simulink model "MCU_Stateflow_Analog"  (R2022b)
settings: Solver=FixedStepDiscrete  StartTime=0.0  StopTime=inf  FixedStep=0.002  RelTol=1e-3
undefined symbols (not defined in the file): ANALOG, cAgeingMode, cCurrentLoopMode, cNoneMode, cParaRecogMode, cSingleBoardMode, cSpeedLoopMode, cTorqueLoopMode, cVvvfOpenMode, FAULT, POWER_ON, STANDBY, TESTBED, VEHICLE, WORKING
libraries: simulink x9, SignalEditorBlockLib x1
(part 1 of 4)
Description:
  | 1、增加Analog模式
  | 2、增加转速选择
settings Model: DataDictionary=MCU_Stateflow_Datadictionary_objects.sldd  Creator=ZYH  LastModifiedBy=ZYH
settings OptimizationCC: DefaultParameterBehavior=Inlined  EnhancedBackFolding=on  PassReuseOutputArgsAs=Individual arguments  ZeroExternalMemoryAtStartup=off  ZeroInternalMemoryAtStartup=off  OptimizeBlockOrder=speed  DifferentSizesBufferReuse=on  OptimizationCustomize=off  EfficientTunableParamExpr=on
settings DebuggingCC: ParameterTunabilityLossMsg=error
settings ModelReferenceCC: ModelReferenceNumInstancesAllowed=Single
settings SFSimCC: MATLABDynamicMemAlloc=off
settings RTWCC: Description=Embedded Coder  SystemTargetFile=ert.tlc  GenCodeOnly=on  TemplateMakefile=ert_default_tmf
settings CodeAppCC: IgnoreCustomStorageClasses=off  OperatorAnnotations=on  SimulinkDataObjDesc=on  SFDataObjDesc=on  CustomSymbolStrGlobalVar=$N$M  CustomSymbolStrType=$N$M_T  CustomSymbolStrFcn=$N$M$F
settings ERTTargetCC: TargetLangStandard=C99 (ISO)  GenerateSampleERTMain=on  InlinedParameterPlacement=NonHierarchical  MultiInstanceErrorCode=None  RootIOFormat=Structure reference  ERTCustomFileTemplate=example_file_process.tlc

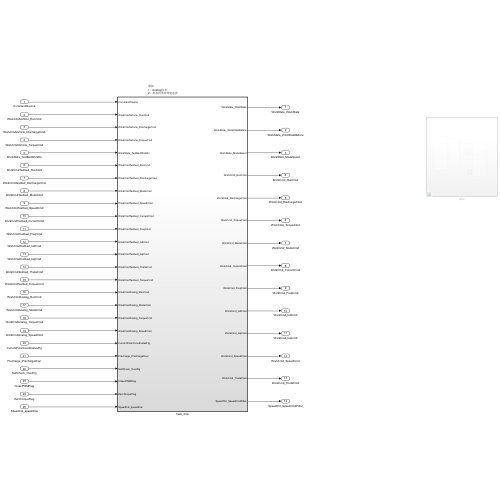
[thumbnail: Simulink's stored preview of the top-level diagram]
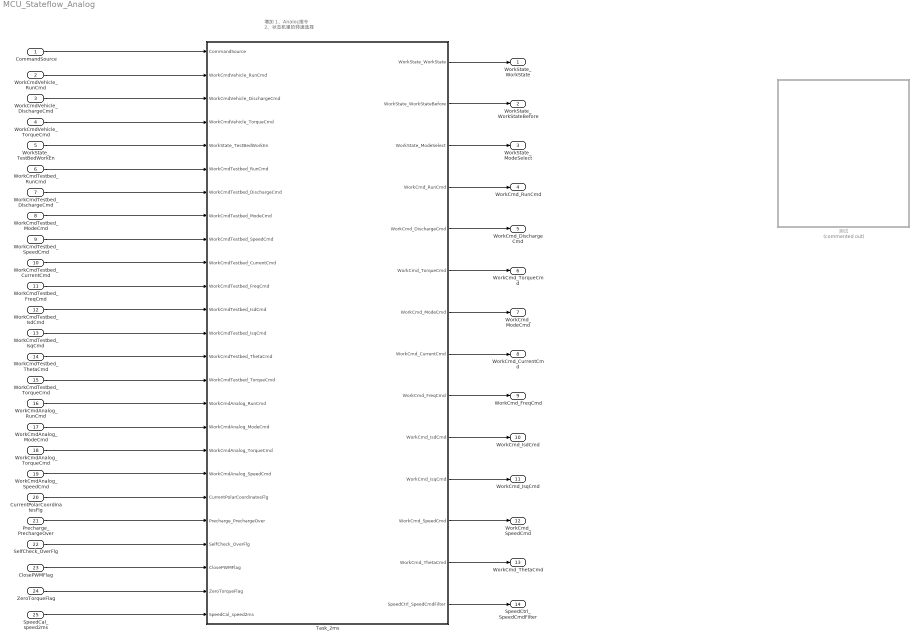
== system MCU_Stateflow_Analog ==
  note: 增加
      | 1、Analog指令
      | 2、状态机里的转速选择
  CommandSource : Inport
  WorkCmdVehicle_RunCmd : Inport  Port=2
  WorkCmdVehicle_DischargeCmd : Inport  Port=3
  WorkCmdVehicle_TorqueCmd : Inport  Port=4
  WorkState_TestBedWorkEn : Inport  Port=5
  WorkCmdTestbed_RunCmd : Inport  Port=6
  WorkCmdTestbed_DischargeCmd : Inport  Port=7
  WorkCmdTestbed_ModeCmd : Inport  Port=8
  WorkCmdTestbed_SpeedCmd : Inport  Port=9
  WorkCmdTestbed_CurrentCmd : Inport  Port=10
  WorkCmdTestbed_FreqCmd : Inport  Port=11
  WorkCmdTestbed_IsdCmd : Inport  Port=12
  WorkCmdTestbed_IsqCmd : Inport  Port=13
  WorkCmdTestbed_ThetaCmd : Inport  Port=14
  WorkCmdTestbed_TorqueCmd : Inport  Port=15
  WorkCmdAnalog_RunCmd : Inport  Port=16
  WorkCmdAnalog_ModeCmd : Inport  Port=17
  WorkCmdAnalog_TorqueCmd : Inport  Port=18
  WorkCmdAnalog_SpeedCmd : Inport  Port=19
  CurrentPolarCoordinatesFlg : Inport  Port=20
  Precharge_PrechargeOver : Inport  Port=21
  SelfCheck_OverFlg : Inport  Port=22
  ClosePWMFlag : Inport  Port=23
  ZeroTorqueFlag : Inport  Port=24
  SpeedCal_speed2ms : Inport  Port=25
  Task_2ms : Subsystem  TreatAsAtomicUnit=on
      settings: RTWSystemCode=Inline
  测试 : Subsystem  Commented=on
  WorkState_WorkState : Outport
  WorkState_WorkStateBefore : Outport  Port=2
  WorkState_ModeSelect : Outport  Port=3
  WorkCmd_RunCmd : Outport  Port=4
  WorkCmd_DischargeCmd : Outport  Port=5
  WorkCmd_TorqueCmd : Outport  Port=6
  WorkCmd_ModeCmd : Outport  Port=7
  WorkCmd_CurrentCmd : Outport  Port=8
  WorkCmd_FreqCmd : Outport  Port=9
  WorkCmd_IsdCmd : Outport  Port=10
  WorkCmd_IsqCmd : Outport  Port=11
  WorkCmd_SpeedCmd : Outport  Port=12
  WorkCmd_ThetaCmd : Outport  Port=13
  SpeedCtrl_SpeedCmdFilter : Outport  Port=14
  wires:
  CommandSource/1 -> Task_2ms/1(CommandSource)
  WorkCmdVehicle_RunCmd/1 -> Task_2ms/2(WorkCmdVehicle_RunCmd)
  WorkCmdVehicle_DischargeCmd/1 -> Task_2ms/3(WorkCmdVehicle_DischargeCmd)
  WorkState_TestBedWorkEn/1 -> Task_2ms/5(WorkState_TestBedWorkEn)
  WorkCmdTestbed_RunCmd/1 -> Task_2ms/6(WorkCmdTestbed_RunCmd)
  WorkCmdTestbed_DischargeCmd/1 -> Task_2ms/7(WorkCmdTestbed_DischargeCmd)
  WorkCmdTestbed_ModeCmd/1 -> Task_2ms/8(WorkCmdTestbed_ModeCmd)
  WorkCmdTestbed_SpeedCmd/1 -> Task_2ms/9(WorkCmdTestbed_SpeedCmd)
  WorkCmdTestbed_CurrentCmd/1 -> Task_2ms/10(WorkCmdTestbed_CurrentCmd)
  WorkCmdTestbed_FreqCmd/1 -> Task_2ms/11(WorkCmdTestbed_FreqCmd)
  WorkCmdTestbed_IsdCmd/1 -> Task_2ms/12(WorkCmdTestbed_IsdCmd)
  WorkCmdTestbed_IsqCmd/1 -> Task_2ms/13(WorkCmdTestbed_IsqCmd)
  WorkCmdTestbed_ThetaCmd/1 -> Task_2ms/14(WorkCmdTestbed_ThetaCmd)
  WorkCmdVehicle_TorqueCmd/1 -> Task_2ms/4(WorkCmdVehicle_TorqueCmd)
  WorkCmdTestbed_TorqueCmd/1 -> Task_2ms/15(WorkCmdTestbed_TorqueCmd)
  CurrentPolarCoordinatesFlg/1 -> Task_2ms/20(CurrentPolarCoordinatesFlg)
  Precharge_PrechargeOver/1 -> Task_2ms/21(Precharge_PrechargeOver)
  ClosePWMFlag/1 -> Task_2ms/23(ClosePWMFlag)
  ZeroTorqueFlag/1 -> Task_2ms/24(ZeroTorqueFlag)
  Task_2ms/1(WorkState_WorkState) -> WorkState_WorkState/1
  Task_2ms/2(WorkState_WorkStateBefore) -> WorkState_WorkStateBefore/1
  Task_2ms/3(WorkState_ModeSelect) -> WorkState_ModeSelect/1
  Task_2ms/4(WorkCmd_RunCmd) -> WorkCmd_RunCmd/1
  Task_2ms/5(WorkCmd_DischargeCmd) -> WorkCmd_DischargeCmd/1
  Task_2ms/6(WorkCmd_TorqueCmd) -> WorkCmd_TorqueCmd/1
  Task_2ms/7(WorkCmd_ModeCmd) -> WorkCmd_ModeCmd/1
  Task_2ms/8(WorkCmd_CurrentCmd) -> WorkCmd_CurrentCmd/1
  Task_2ms/9(WorkCmd_FreqCmd) -> WorkCmd_FreqCmd/1
  Task_2ms/10(WorkCmd_IsdCmd) -> WorkCmd_IsdCmd/1
  Task_2ms/11(WorkCmd_IsqCmd) -> WorkCmd_IsqCmd/1
  Task_2ms/12(WorkCmd_SpeedCmd) -> WorkCmd_SpeedCmd/1
  Task_2ms/13(WorkCmd_ThetaCmd) -> WorkCmd_ThetaCmd/1
  SelfCheck_OverFlg/1 -> Task_2ms/22(SelfCheck_OverFlg)
  WorkCmdAnalog_RunCmd/1 -> Task_2ms/16(WorkCmdAnalog_RunCmd)
  WorkCmdAnalog_ModeCmd/1 -> Task_2ms/17(WorkCmdAnalog_ModeCmd)
  WorkCmdAnalog_TorqueCmd/1 -> Task_2ms/18(WorkCmdAnalog_TorqueCmd)
  WorkCmdAnalog_SpeedCmd/1 -> Task_2ms/19(WorkCmdAnalog_SpeedCmd)
  SpeedCal_speed2ms/1 -> Task_2ms/25(SpeedCal_speed2ms)
  Task_2ms/14(SpeedCtrl_SpeedCmdFilter) -> SpeedCtrl_SpeedCmdFilter/1

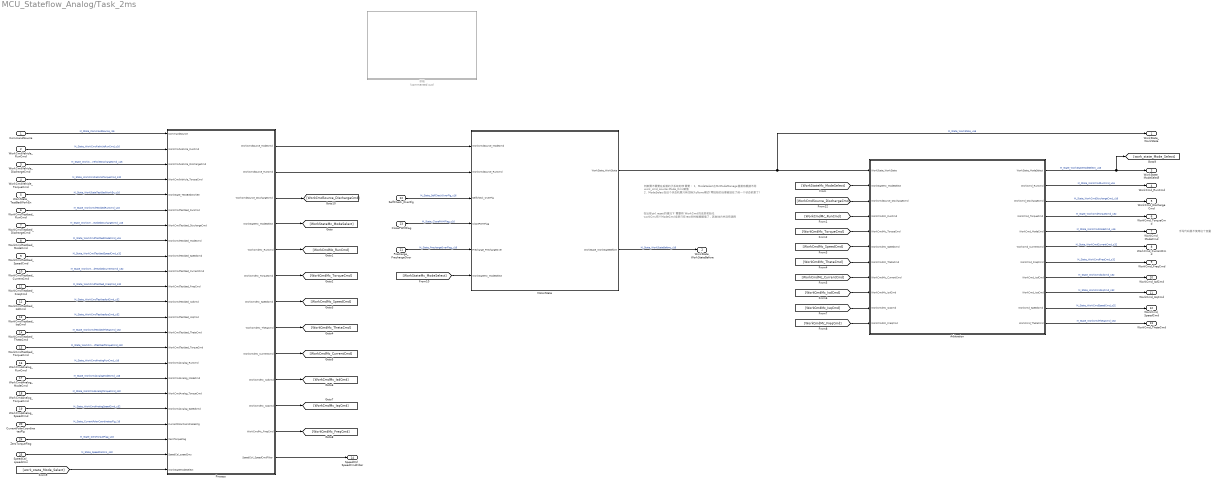
== system MCU_Stateflow_Analog/Task_2ms ==
  note: 手写代码里不使用这个变量
  note: 在出现ctrl_reset的情况下
      | 需要将 WorkCmd 的成员初始化
      | workCmd有个ModeCmd成员只在rest的时候被赋值了，其他地方并没有调用
  note: 判断需不需要在后面的子系统处理
      |
      | 需要：
      | 1、ModeSelect在McModeManage里面有根据不同 work_cmd_source.Mode_Cmd赋值
      | 2、ModeSelect在这个状态机里只有切换为cNone模式(零扭矩的处理被放在了前一个状态机里了)
  CommandSource : Inport
  WorkCmdVehicle_RunCmd : Inport  Port=2
  WorkCmdVehicle_DischargeCmd : Inport  Port=3
  WorkCmdVehicle_TorqueCmd : Inport  Port=4
  WorkState_TestBedWorkEn : Inport  Port=5
  WorkCmdTestbed_RunCmd : Inport  Port=6
  WorkCmdTestbed_DischargeCmd : Inport  Port=7
  WorkCmdTestbed_ModeCmd : Inport  Port=8
  WorkCmdTestbed_SpeedCmd : Inport  Port=9
  WorkCmdTestbed_CurrentCmd : Inport  Port=10
  WorkCmdTestbed_FreqCmd : Inport  Port=11
  WorkCmdTestbed_IsdCmd : Inport  Port=12
  WorkCmdTestbed_IsqCmd : Inport  Port=13
  WorkCmdTestbed_ThetaCmd : Inport  Port=14
  WorkCmdTestbed_TorqueCmd : Inport  Port=15
  WorkCmdAnalog_RunCmd : Inport  Port=16
  WorkCmdAnalog_ModeCmd : Inport  Port=17
  WorkCmdAnalog_TorqueCmd : Inport  Port=18
  WorkCmdAnalog_SpeedCmd : Inport  Port=19
  CurrentPolarCoordinatesFlg : Inport  Port=20
  Precharge_PrechargeOver : Inport  Port=21
  SelfCheck_OverFlg : Inport  Port=22
  ClosePWMFlag : Inport  Port=23
  ZeroTorqueFlag : Inport  Port=24
  SpeedCal_speed2ms : Inport  Port=25
  Arbitration : Subsystem  TreatAsAtomicUnit=on
  MotorState : Stateflow chart  TreatAsAtomicUnit=on
      settings: RTWSystemCode=Reusable function  PortSchema="{\"entries\":[{\"content\":{\"sides\":[{\"content\":{\"connectorIds\":[\"In4\",\"In3\",\"In1\",\"In2\",\"In5\",\"In6\"]},\"type\":\"ConnectorPlacement.EquallySpacedRectSide\",\"uuid\":\"e0adab7d-9c82-44fd-b38c-331bb9d71454\"},{\"content\":{\"connectorIds\":[\"Out1\",\"Out2\"],\"side\":\"RIGHT\"},\"type\":\"ConnectorPlacement.EquallySpacedRectSide\",\"uuid\":\"98ad1acc-debf-46f0-91aa-4bd2062f60b6\"},{\"content\":{\"connectorIds\":[],\"side\":\"TOP\"},\"type\":\"ConnectorPlacement.EquallySpacedRectSide\",\"uuid\":\"a7c2d312-245c-4ce1-bea5-1bac95c515f1\"},{\"content\":{\"connectorIds\":[],\"side\":\"BOTTOM\"},\"type\":\"ConnectorPlacement.EquallySpacedRectSide\",\"uuid\":\"175f3b6b-1019-4e6e-83d9-bf4c82f74bc8\"}]},\"type\":\"ConnectorPlacement.EquallySpacedConnector\",\"uuid\":\"df312d8c-c57e-4b1a-958b-330641c1b4d1\"}],\"packageUris\":[\"http://schema.mathworks.com/mf0/Connector/R2020b\"],\"version\":\"1.0\"}"
  Process : Subsystem  TreatAsAtomicUnit=on
  草稿 : Subsystem  Commented=on
  WorkState_WorkState : Outport
  WorkState_WorkStateBefore : Outport  Port=2
  WorkState_ModeSelect : Outport  Port=3
  WorkCmd_RunCmd : Outport  Port=4
  WorkCmd_DischargeCmd : Outport  Port=5
  WorkCmd_TorqueCmd : Outport  Port=6
  WorkCmd_ModeCmd : Outport  Port=7
  WorkCmd_CurrentCmd : Outport  Port=8
  WorkCmd_FreqCmd : Outport  Port=9
  WorkCmd_IsdCmd : Outport  Port=10
  WorkCmd_IsqCmd : Outport  Port=11
  WorkCmd_SpeedCmd : Outport  Port=12
  WorkCmd_ThetaCmd : Outport  Port=13
  SpeedCtrl_SpeedCmdFilter : Outport  Port=14
  wires:
  MotorState/1(WorkState_WorkState) -> WorkState_WorkState/1, Arbitration/1(WorkState_WorkState)  "M_State_WorkState_u16"
  [WorkStateMc_ModeSelect] -> Arbitration/2(WorkStateMc_ModeSelect)
  [WorkCmdMc_RunCmd] -> Arbitration/4(WorkCmdMc_RunCmd)
  [WorkCmdMc_TorqueCmd] -> Arbitration/5(WorkCmdMc_TorqueCmd)
  [WorkCmdMc_SpeedCmd] -> Arbitration/6(WorkCmdMc_SpeedCmd)
  [WorkCmdMc_ThetaCmd] -> Arbitration/7(WorkCmdMc_ThetaCmd)
  [WorkCmdMc_CurrentCmd] -> Arbitration/8(WorkCmdMc_CurrentCmd)
  [WorkCmdMc_IsdCmd] -> Arbitration/9(WorkCmdMc_IsdCmd)
  [WorkCmdMc_IsqCmd] -> Arbitration/10(WorkCmdMc_IsqCmd)
  [WorkCmdMc_FreqCmd] -> Arbitration/11(WorkCmdMc_FreqCmd)
  Precharge_PrechargeOver/1 -> MotorState/5(Precharge_PrechargeOver)  "M_State_PrechargeOverFlag_u16"
  MotorState/2(WorkState_WorkStateBefore) -> WorkState_WorkStateBefore/1  "M_State_WorkStateBefore_u16"
  Process/8(WorkCmdMc_ThetaCmd) -> [WorkCmdMc_ThetaCmd]
  Process/9(WorkCmdMc_CurrentCmd) -> [WorkCmdMc_CurrentCmd]
  Process/7(WorkCmdMc_SpeedCmd) -> [WorkCmdMc_SpeedCmd]
  Process/12(WorkCmdMc_FreqCmd) -> [WorkCmdMc_FreqCmd]
  Process/5(WorkCmdMc_RunCmd) -> [WorkCmdMc_RunCmd]
  Process/10(WorkCmdMc_IsdCmd) -> [WorkCmdMc_IsdCmd]
  Process/11(WorkCmdMc_IsqCmd) -> [WorkCmdMc_IsqCmd]
  Process/6(WorkCmdMc_TorqueCmd) -> [WorkCmdMc_TorqueCmd]
  Process/4(WorkStateMc_ModeSelect) -> [WorkStateMc_ModeSelect]
  CommandSource/1 -> Process/1(CommandSource)  "M_State_CommandSource_i16"
  WorkCmdVehicle_RunCmd/1 -> Process/2(WorkCmdVehicle_RunCmd)  "M_State_WorkCmdVehicleRunCmd_u16"
  WorkCmdVehicle_DischargeCmd/1 -> Process/3(WorkCmdVehicle_DischargeCmd)  "M_State_WorkCmdVehicleDischargeCmd_u16"
  WorkState_TestBedWorkEn/1 -> Process/5(WorkState_TestBedWorkEn)  "M_State_WorkStateTestBedWorkEn_u16"
  WorkCmdTestbed_RunCmd/1 -> Process/6(WorkCmdTestbed_RunCmd)  "M_State_WorkCmdTestbedRunCmd_u16"
  WorkCmdTestbed_DischargeCmd/1 -> Process/7(WorkCmdTestbed_DischargeCmd)  "M_State_WorkCmdTestbedDischargeCmd_u16"
  WorkCmdTestbed_ModeCmd/1 -> Process/8(WorkCmdTestbed_ModeCmd)  "M_State_WorkCmdTestbedModeCmd_u16"
  WorkCmdTestbed_SpeedCmd/1 -> Process/9(WorkCmdTestbed_SpeedCmd)  "M_State_WorkCmdTestbedSpeedCmd_s32"
  WorkCmdTestbed_CurrentCmd/1 -> Process/10(WorkCmdTestbed_CurrentCmd)  "M_State_WorkCmdTestbedCurrentCmd_s32"
  WorkCmdTestbed_FreqCmd/1 -> Process/11(WorkCmdTestbed_FreqCmd)  "M_State_WorkCmdTestbed_FreqCmd_s32"
  WorkCmdTestbed_IsdCmd/1 -> Process/12(WorkCmdTestbed_IsdCmd)  "M_State_WorkCmdTestbedIsdCmd_s32"
  WorkCmdTestbed_IsqCmd/1 -> Process/13(WorkCmdTestbed_IsqCmd)  "M_State_WorkCmdTestbedIsqCmd_s32"
  WorkCmdTestbed_ThetaCmd/1 -> Process/14(WorkCmdTestbed_ThetaCmd)  "M_State_WorkCmdTestbedThetaCmd_s32"
  WorkCmdVehicle_TorqueCmd/1 -> Process/4(WorkCmdVehicle_TorqueCmd)  "M_State_WorkCmdVehicleTorqueCmd_s32"
  WorkCmdTestbed_TorqueCmd/1 -> Process/15(WorkCmdTestbed_TorqueCmd)  "M_State_WorkCmdTestbedTorqueCmd_s32"
  CurrentPolarCoordinatesFlg/1 -> Process/20(CurrentPolarCoordinatesFlg)  "M_State_CurrentPolarCoordinatesFlg_i16"
  ZeroTorqueFlag/1 -> Process/21(ZeroTorqueFlag)  "M_State_ZeroTorqueFlag_u16"
  Process/1(WorkCmdSource_ModeCmd) -> MotorState/4(WorkCmdSource_ModeCmd)
  Process/2(WorkCmdSource_RunCmd) -> MotorState/3(WorkCmdSource_RunCmd)
  Arbitration/1(WorkState_ModeSelect) -> WorkState_ModeSelect/1, [work_state_Mode_Select]  "M_State_WorkStateModeSelect_u16"
  Arbitration/2(WorkCmd_RunCmd) -> WorkCmd_RunCmd/1  "M_State_WorkCmdRunCmd_u16"
  Arbitration/3(WorkCmd_DischargeCmd) -> WorkCmd_DischargeCmd/1  "M_State_WorkCmdDischargeCmd_u16"
  Arbitration/4(WorkCmd_TorqueCmd) -> WorkCmd_TorqueCmd/1  "M_State_WorkCmdTorqueCmd_s32"
  Arbitration/5(WorkCmd_ModeCmd) -> WorkCmd_ModeCmd/1  "M_State_WorkCmdModeCmd_u16"
  Arbitration/6(WorkCmd_CurrentCmd) -> WorkCmd_CurrentCmd/1  "M_State_WorkCmdCurrentCmd_s32"
  Arbitration/7(WorkCmd_FreqCmd) -> WorkCmd_FreqCmd/1  "M_State_WorkCmdFreqCmd_s32"
  Arbitration/8(WorkCmd_IsdCmd) -> WorkCmd_IsdCmd/1  "M_State_WorkCmdIsdCmd_s32"
  Arbitration/9(WorkCmd_IsqCmd) -> WorkCmd_IsqCmd/1  "M_State_WorkCmdIsqCmd_s32"
  Arbitration/10(WorkCmd_SpeedCmd) -> WorkCmd_SpeedCmd/1  "M_State_WorkCmdSpeedCmd_s32"
  Arbitration/11(WorkCmd_ThetaCmd) -> WorkCmd_ThetaCmd/1  "M_State_WorkCmdThetaCmd_s32"
  SelfCheck_OverFlg/1 -> MotorState/1(SelfCheck_OverFlg)  "M_State_SelfCheckOverFlg_u16"
  ClosePWMFlag/1 -> MotorState/2(ClosePWMFlag)  "M_State_ClosePWMFlag_u16"
  [work_state_Mode_Select] -> Process/23(WorkStateModeSelect)
  [WorkStateMc_ModeSelect] -> MotorState/6(WorkStateMc_ModeSelect)
  WorkCmdAnalog_RunCmd/1 -> Process/16(WorkCmdAnalog_RunCmd)  "M_State_WorkCmdAnalogRunCmd_u16"
  WorkCmdAnalog_ModeCmd/1 -> Process/17(WorkCmdAnalog_ModeCmd)  "M_State_WorkCmdAnalogModeCmd_u16"
  WorkCmdAnalog_TorqueCmd/1 -> Process/18(WorkCmdAnalog_TorqueCmd)  "M_State_WorkCmdAnalogTorqueCmd_s32"
  WorkCmdAnalog_SpeedCmd/1 -> Process/19(WorkCmdAnalog_SpeedCmd)  "M_State_WorkCmdAnalogSpeedCmd_s32"
  SpeedCal_speed2ms/1 -> Process/22(SpeedCal_speed2ms)  "M_State_SpeedCal2ms_s32"
  Process/13(SpeedCtrl_SpeedCmdFilter) -> SpeedCtrl_SpeedCmdFilter/1
  Process/3(WorkCmdSource_DischargeCmd) -> [WorkCmdSource_DischargeCmd]
  [WorkCmdSource_DischargeCmd] -> Arbitration/3(WorkCmdSource_DischargeCmd)

== system MCU_Stateflow_Analog/测试 ==
  Constant : Constant  Commented=on
  Constant1 : Constant  Commented=on  Value=0
  Constant2 : Constant  Commented=on  Value=2
  Constant3 : Constant  Commented=on  Value=200
  Constant4 : Constant  Commented=on
  Constant5 : Constant  Commented=on  Value=0
  Data Type Conversion{,1..5} (6 alike) : DataTypeConversion  Commented=on  SaturateOnIntegerOverflow=off  RndMeth=Floor
  Display : Display  Commented=on
  Display1 : Display  Commented=on
  Signal Editor : SignalEditorBlockLib/Signal Editor  Commented=on  FileName=Inputs.mat  ActiveScenario=Scenario  ActiveSignal=CommandSource  IsBus=off  OutputBusObjectStr=Bus: BusObject  SampleTime=0  Interpolate=off  ZeroCross=off  OutputAfterFinalValue=Setting to zero  Unit=inherit  PreserveSignalName=on
  Task_2ms1 : Subsystem  Commented=on  TreatAsAtomicUnit=on
      settings: RTWSystemCode=Inline
  Task_2ms2 : Subsystem  Commented=on  TreatAsAtomicUnit=on
      settings: RTWSystemCode=Inline
  wires:
  Constant/1 -> Data Type Conversion/1
  Constant3/1 -> Data Type Conversion3/1
  Task_2ms1/1(WorkState_WorkState) -> Display/1
  Data Type Conversion5/1 -> Task_2ms1/24(ZeroTorqueFlag), Task_2ms1/23(ClosePWMFlag)
  Data Type Conversion2/1 -> Task_2ms1/8(WorkCmdTestbed_ModeCmd)
  Data Type Conversion4/1 -> Task_2ms1/22(SelfCheck_OverFlg), Task_2ms1/21(Precharge_PrechargeOver)
  Data Type Conversion3/1 -> Task_2ms1/9(WorkCmdTestbed_SpeedCmd)
  Task_2ms1/12(WorkCmd_SpeedCmd) -> Display1/1
  Constant5/1 -> Data Type Conversion5/1
  Constant4/1 -> Data Type Conversion4/1
  Data Type Conversion1/1 -> Task_2ms1/6(WorkCmdTestbed_RunCmd), Task_2ms1/5(WorkState_TestBedWorkEn)
  Constant1/1 -> Data Type Conversion1/1
  Constant2/1 -> Data Type Conversion2/1
  Data Type Conversion/1 -> Task_2ms1/1(CommandSource)

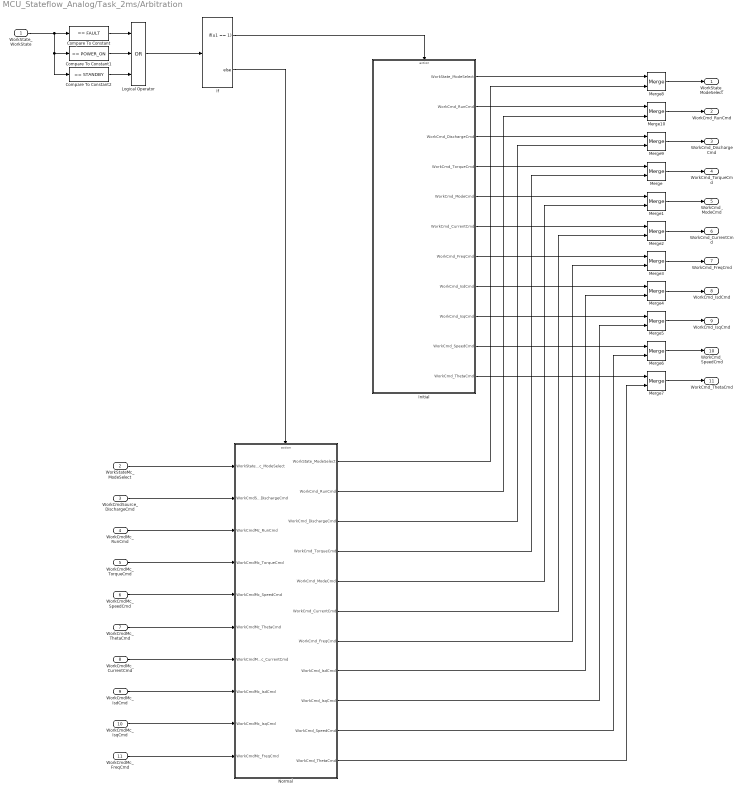
== system MCU_Stateflow_Analog/Task_2ms/Arbitration ==
  WorkState_WorkState : Inport
  WorkStateMc_ModeSelect : Inport  Port=2
  WorkCmdSource_DischargeCmd : Inport  Port=3
  WorkCmdMc_RunCmd : Inport  Port=4
  WorkCmdMc_TorqueCmd : Inport  Port=5
  WorkCmdMc_SpeedCmd : Inport  Port=6
  WorkCmdMc_ThetaCmd : Inport  Port=7
  WorkCmdMc_CurrentCmd : Inport  Port=8
  WorkCmdMc_IsdCmd : Inport  Port=9
  WorkCmdMc_IsqCmd : Inport  Port=10
  WorkCmdMc_FreqCmd : Inport  Port=11
  Compare To Constant : simulink/Logic and Bit Operations/Compare To Constant  relop===  const=FAULT  OutDataTypeStr=boolean
  Compare To Constant1 : simulink/Logic and Bit Operations/Compare To Constant  relop===  const=POWER_ON  OutDataTypeStr=boolean
  Compare To Constant2 : simulink/Logic and Bit Operations/Compare To Constant  relop===  const=STANDBY  OutDataTypeStr=boolean
  If : If  IfExpression=u1 == 1
  Initial : Subsystem  TreatAsAtomicUnit=on
  Logical Operator : Logic  Operator=OR  Inputs=3  AllPortsSameDT=off  OutDataTypeStr=boolean
  Merge{,1..10} (11 alike) : Merge
  Normal : Subsystem  TreatAsAtomicUnit=on
  WorkState_ModeSelect : Outport
  WorkCmd_RunCmd : Outport  Port=2
  WorkCmd_DischargeCmd : Outport  Port=3
  WorkCmd_TorqueCmd : Outport  Port=4
  WorkCmd_ModeCmd : Outport  Port=5
  WorkCmd_CurrentCmd : Outport  Port=6
  WorkCmd_FreqCmd : Outport  Port=7
  WorkCmd_IsdCmd : Outport  Port=8
  WorkCmd_IsqCmd : Outport  Port=9
  WorkCmd_SpeedCmd : Outport  Port=10
  WorkCmd_ThetaCmd : Outport  Port=11
  wires:
  WorkState_WorkState/1 -> Compare To Constant2/1, Compare To Constant1/1, Compare To Constant/1
  Compare To Constant/1 -> Logical Operator/1
  Compare To Constant1/1 -> Logical Operator/2
  Compare To Constant2/1 -> Logical Operator/3
  Logical Operator/1 -> If/1
  If/1 -> Initial/Action
  If/2 -> Normal/Action
  Initial/11(WorkCmd_ThetaCmd) -> Merge7/1
  Initial/10(WorkCmd_SpeedCmd) -> Merge6/1
  Initial/9(WorkCmd_IsqCmd) -> Merge5/1
  Initial/8(WorkCmd_IsdCmd) -> Merge4/1
  Initial/7(WorkCmd_FreqCmd) -> Merge3/1
  Initial/6(WorkCmd_CurrentCmd) -> Merge2/1
  Initial/5(WorkCmd_ModeCmd) -> Merge1/1
  Initial/4(WorkCmd_TorqueCmd) -> Merge/1
  Initial/3(WorkCmd_DischargeCmd) -> Merge9/1
  WorkStateMc_ModeSelect/1 -> Normal/1(WorkStateMc_ModeSelect)
  WorkCmdMc_RunCmd/1 -> Normal/3(WorkCmdMc_RunCmd)
  WorkCmdMc_TorqueCmd/1 -> Normal/4(WorkCmdMc_TorqueCmd)
  WorkCmdMc_SpeedCmd/1 -> Normal/5(WorkCmdMc_SpeedCmd)
  WorkCmdMc_ThetaCmd/1 -> Normal/6(WorkCmdMc_ThetaCmd)
  WorkCmdMc_CurrentCmd/1 -> Normal/7(WorkCmdMc_CurrentCmd)
  WorkCmdMc_IsdCmd/1 -> Normal/8(WorkCmdMc_IsdCmd)
  WorkCmdMc_IsqCmd/1 -> Normal/9(WorkCmdMc_IsqCmd)
  WorkCmdMc_FreqCmd/1 -> Normal/10(WorkCmdMc_FreqCmd)
  Merge/1 -> WorkCmd_TorqueCmd/1
  Merge1/1 -> WorkCmd_ModeCmd/1
  Merge2/1 -> WorkCmd_CurrentCmd/1
  Merge3/1 -> WorkCmd_FreqCmd/1
  Merge4/1 -> WorkCmd_IsdCmd/1
  Merge5/1 -> WorkCmd_IsqCmd/1
  Merge6/1 -> WorkCmd_SpeedCmd/1
  Merge7/1 -> WorkCmd_ThetaCmd/1
  Initial/1(WorkState_ModeSelect) -> Merge8/1
  Merge8/1 -> WorkState_ModeSelect/1
  Initial/2(WorkCmd_RunCmd) -> Merge10/1
  Merge10/1 -> WorkCmd_RunCmd/1
  Merge9/1 -> WorkCmd_DischargeCmd/1
  Normal/1(WorkState_ModeSelect) -> Merge8/2
  Normal/2(WorkCmd_RunCmd) -> Merge10/2
  Normal/3(WorkCmd_DischargeCmd) -> Merge9/2
  Normal/4(WorkCmd_TorqueCmd) -> Merge/2
  Normal/5(WorkCmd_ModeCmd) -> Merge1/2
  Normal/6(WorkCmd_CurrentCmd) -> Merge2/2
  Normal/7(WorkCmd_FreqCmd) -> Merge3/2
  Normal/8(WorkCmd_IsdCmd) -> Merge4/2
  Normal/9(WorkCmd_IsqCmd) -> Merge5/2
  Normal/10(WorkCmd_SpeedCmd) -> Merge6/2
  Normal/11(WorkCmd_ThetaCmd) -> Merge7/2
  WorkCmdSource_DischargeCmd/1 -> Normal/2(WorkCmdSource_DischargeCmd)

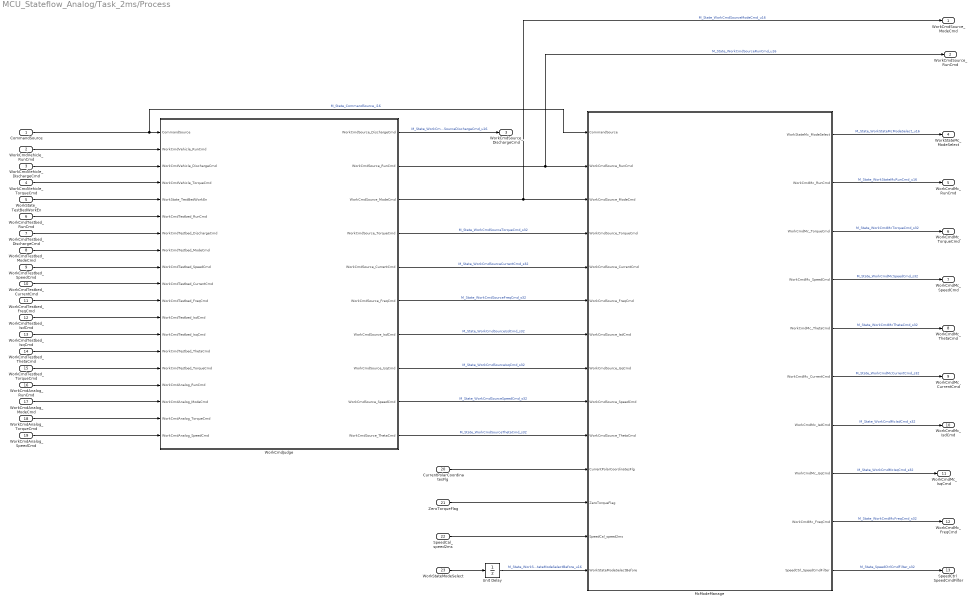
== system MCU_Stateflow_Analog/Task_2ms/Process ==
  CommandSource : Inport
  WorkCmdVehicle_RunCmd : Inport  Port=2
  WorkCmdVehicle_DischargeCmd : Inport  Port=3
  WorkCmdVehicle_TorqueCmd : Inport  Port=4
  WorkState_TestBedWorkEn : Inport  Port=5
  WorkCmdTestbed_RunCmd : Inport  Port=6
  WorkCmdTestbed_DischargeCmd : Inport  Port=7
  WorkCmdTestbed_ModeCmd : Inport  Port=8
  WorkCmdTestbed_SpeedCmd : Inport  Port=9
  WorkCmdTestbed_CurrentCmd : Inport  Port=10
  WorkCmdTestbed_FreqCmd : Inport  Port=11
  WorkCmdTestbed_IsdCmd : Inport  Port=12
  WorkCmdTestbed_IsqCmd : Inport  Port=13
  WorkCmdTestbed_ThetaCmd : Inport  Port=14
  WorkCmdTestbed_TorqueCmd : Inport  Port=15
  WorkCmdAnalog_RunCmd : Inport  Port=16
  WorkCmdAnalog_ModeCmd : Inport  Port=17
  WorkCmdAnalog_TorqueCmd : Inport  Port=18
  WorkCmdAnalog_SpeedCmd : Inport  Port=19
  CurrentPolarCoordinatesFlg : Inport  Port=20
  ZeroTorqueFlag : Inport  Port=21
  SpeedCal_speed2ms : Inport  Port=22
  WorkStateModeSelect : Inport  Port=23
  McModeManage : Stateflow chart  TreatAsAtomicUnit=on
      settings: RTWSystemCode=Reusable function  FunctionInterfaceSpec=Allow arguments (Optimized)  PortSchema="{\"entries\":[{\"content\":{\"sides\":[{\"content\":{\"connectorIds\":[\"In2\",\"In4\",\"In3\",\"In5\",\"In6\",\"In7\",\"In8\",\"In9\",\"In10\",\"In1\",\"In11\",\"In12\",\"In13\",\"In14\"]},\"type\":\"ConnectorPlacement.EquallySpacedRectSide\",\"uuid\":\"2e7d3842-0a61-4590-9292-7a5bc1b6d63e\"},{\"content\":{\"connectorIds\":[\"Out1\",\"Out2\",\"Out3\",\"Out4\",\"Out5\",\"Out6\",\"Out7\",\"Out8\",\"Out9\",\"Out10\"],\"side\":\"RIGHT\"},\"type\":\"ConnectorPlacement.EquallySpacedRectSide\",\"uuid\":\"fb66f02a-321f-47a6-a489-4b94442e22c8\"},{\"content\":{\"connectorIds\":[],\"side\":\"TOP\"},\"type\":\"ConnectorPlacement.EquallySpacedRectSide\",\"uuid\":\"26cfdcf8-827e-48d9-aa42-40739db869be\"},{\"content\":{\"connectorIds\":[],\"side\":\"BOTTOM\"},\"type\":\"ConnectorPlacement.EquallySpacedRectSide\",\"uuid\":\"3bc2be8d-756f-48d1-976e-919451ea6fa2\"}]},\"type\":\"ConnectorPlacement.EquallySpacedConnector\",\"uuid\":\"eb156a25-beb1-4594-a414-e9203ec852c3\"}],\"packageUris\":[\"http://schema.mathworks.com/mf0/Connector/R2020b\"],\"version\":\"1.0\"}"
  Unit Delay : UnitDelay  SampleTime=-1  HasFrameUpgradeWarning=on
  WorkCmdJudge : Stateflow chart  TreatAsAtomicUnit=on
      settings: RTWSystemCode=Reusable function  FunctionInterfaceSpec=Allow arguments (Optimized)  PortSchema="{\"entries\":[{\"content\":{\"sides\":[{\"content\":{\"connectorIds\":[\"In2\",\"In3\",\"In4\",\"In15\",\"In5\",\"In6\",\"In7\",\"In8\",\"In9\",\"In10\",\"In11\",\"In12\",\"In13\",\"In14\",\"In16\",\"In17\",\"In1\",\"In19\",\"In18\"]},\"type\":\"ConnectorPlacement.EquallySpacedRectSide\",\"uuid\":\"08f79912-2405-4f04-9254-689ee53f44b9\"},{\"content\":{\"connectorIds\":[\"Out1\",\"Out2\",\"Out3\",\"Out10\",\"Out4\",\"Out5\",\"Out6\",\"Out7\",\"Out8\",\"Out9\"],\"side\":\"RIGHT\"},\"type\":\"ConnectorPlacement.EquallySpacedRectSide\",\"uuid\":\"8406ee0b-fe03-429b-8d11-a315759dccf9\"},{\"content\":{\"connectorIds\":[],\"side\":\"TOP\"},\"type\":\"ConnectorPlacement.EquallySpacedRectSide\",\"uuid\":\"82a87416-6ee6-4a7e-925f-181c5fe86ae8\"},{\"content\":{\"connectorIds\":[],\"side\":\"BOTTOM\"},\"type\":\"ConnectorPlacement.EquallySpacedRectSide\",\"uuid\":\"850ffd8e-4d4e-428c-999d-6858cee77358\"}]},\"type\":\"ConnectorPlacement.EquallySpacedConnector\",\"uuid\":\"ba5e9ad6-4f64-4c0c-82e6-bf977e3fd6e6\"}],\"packageUris\":[\"http://schema.mathworks.com/mf0/Connector/R2020b\"],\"version\":\"1.0\"}"
  WorkCmdSource_ModeCmd : Outport
  WorkCmdSource_RunCmd : Outport  Port=2
  WorkCmdSource_DischargeCmd : Outport  Port=3
  WorkStateMc_ModeSelect : Outport  Port=4
  WorkCmdMc_RunCmd : Outport  Port=5
  WorkCmdMc_TorqueCmd : Outport  Port=6
  WorkCmdMc_SpeedCmd : Outport  Port=7
  WorkCmdMc_ThetaCmd : Outport  Port=8
  WorkCmdMc_CurrentCmd : Outport  Port=9
  WorkCmdMc_IsdCmd : Outport  Port=10
  WorkCmdMc_IsqCmd : Outport  Port=11
  WorkCmdMc_FreqCmd : Outport  Port=12
  SpeedCtrl_SpeedCmdFilter : Outport  Port=13
  wires:
  WorkCmdJudge/8(WorkCmdSource_SpeedCmd) -> McModeManage/10(WorkCmdSource_SpeedCmd)  "M_State_WorkCmdSourceSpeedCmd_s32"
  CommandSource/1 -> WorkCmdJudge/2(CommandSource), McModeManage/2(CommandSource)  "M_State_CommandSource_i16"
  WorkCmdJudge/4(WorkCmdSource_CurrentCmd) -> McModeManage/6(WorkCmdSource_CurrentCmd)  "M_State_WorkCmdSourceCurrentCmd_s32"
  WorkCmdJudge/6(WorkCmdSource_IsdCmd) -> McModeManage/8(WorkCmdSource_IsdCmd)  "M_State_WorkCmdSourceIsdCmd_s32"
  WorkCmdJudge/2(WorkCmdSource_RunCmd) -> WorkCmdSource_RunCmd/1, McModeManage/4(WorkCmdSource_RunCmd)  "M_State_WorkCmdSourceRunCmd_u16"
  WorkCmdTestbed_ThetaCmd/1 -> WorkCmdJudge/14(WorkCmdTestbed_ThetaCmd)
  WorkCmdJudge/7(WorkCmdSource_IsqCmd) -> McModeManage/9(WorkCmdSource_IsqCmd)  "M_State_WorkCmdSourceIsqCmd_s32"
  McModeManage/9(WorkCmdMc_FreqCmd) -> WorkCmdMc_FreqCmd/1  "M_State_WorkCmdMcFreqCmd_s32"
  McModeManage/2(WorkCmdMc_RunCmd) -> WorkCmdMc_RunCmd/1  "M_State_WorkStateMcRunCmd_u16"
  WorkCmdJudge/5(WorkCmdSource_FreqCmd) -> McModeManage/7(WorkCmdSource_FreqCmd)  "M_State_WorkCmdSourceFreqCmd_s32"
  WorkCmdJudge/10(WorkCmdSource_TorqueCmd) -> McModeManage/5(WorkCmdSource_TorqueCmd)  "M_State_WorkCmdSourceTorqueCmd_s32"
  McModeManage/4(WorkCmdMc_SpeedCmd) -> WorkCmdMc_SpeedCmd/1  "M_State_WorkCmdMcSpeedCmd_s32"
  WorkCmdJudge/9(WorkCmdSource_ThetaCmd) -> McModeManage/1(WorkCmdSource_ThetaCmd)  "M_State_WorkCmdSourceThetaCmd_s32"
  WorkCmdVehicle_RunCmd/1 -> WorkCmdJudge/3(WorkCmdVehicle_RunCmd)
  WorkCmdTestbed_IsdCmd/1 -> WorkCmdJudge/12(WorkCmdTestbed_IsdCmd)
  WorkCmdTestbed_IsqCmd/1 -> WorkCmdJudge/13(WorkCmdTestbed_IsqCmd)
  WorkCmdJudge/1(WorkCmdSource_DischargeCmd) -> WorkCmdSource_DischargeCmd/1  "M_State_WorkCmdSourceDischargeCmd_u16"
  McModeManage/1(WorkStateMc_ModeSelect) -> WorkStateMc_ModeSelect/1  "M_State_WorkStateMcModeSelect_u16"
  WorkCmdTestbed_TorqueCmd/1 -> WorkCmdJudge/16(WorkCmdTestbed_TorqueCmd)
  WorkCmdJudge/3(WorkCmdSource_ModeCmd) -> WorkCmdSource_ModeCmd/1, McModeManage/3(WorkCmdSource_ModeCmd)  "M_State_WorkCmdSourceModeCmd_u16"
  WorkCmdTestbed_ModeCmd/1 -> WorkCmdJudge/8(WorkCmdTestbed_ModeCmd)
  WorkCmdTestbed_DischargeCmd/1 -> WorkCmdJudge/7(WorkCmdTestbed_DischargeCmd)
  WorkCmdTestbed_RunCmd/1 -> WorkCmdJudge/6(WorkCmdTestbed_RunCmd)
  WorkCmdVehicle_DischargeCmd/1 -> WorkCmdJudge/4(WorkCmdVehicle_DischargeCmd)
  WorkCmdVehicle_TorqueCmd/1 -> WorkCmdJudge/15(WorkCmdVehicle_TorqueCmd)
  WorkState_TestBedWorkEn/1 -> WorkCmdJudge/5(WorkState_TestBedWorkEn)
  WorkCmdTestbed_CurrentCmd/1 -> WorkCmdJudge/10(WorkCmdTestbed_CurrentCmd)
  McModeManage/6(WorkCmdMc_CurrentCmd) -> WorkCmdMc_CurrentCmd/1  "M_State_WorkCmdMcCurrentCmd_s32"
  McModeManage/5(WorkCmdMc_ThetaCmd) -> WorkCmdMc_ThetaCmd/1  "M_State_WorkCmdMcThetaCmd_s32"
  McModeManage/7(WorkCmdMc_IsdCmd) -> WorkCmdMc_IsdCmd/1  "M_State_WorkCmdMcIsdCmd_s32"
  WorkCmdTestbed_SpeedCmd/1 -> WorkCmdJudge/9(WorkCmdTestbed_SpeedCmd)
  McModeManage/3(WorkCmdMc_TorqueCmd) -> WorkCmdMc_TorqueCmd/1  "M_State_WorkCmdMcTorqueCmd_s32"
  McModeManage/8(WorkCmdMc_IsqCmd) -> WorkCmdMc_IsqCmd/1  "M_State_WorkCmdMcIsqCmd_s32"
  WorkCmdTestbed_FreqCmd/1 -> WorkCmdJudge/11(WorkCmdTestbed_FreqCmd)
  WorkStateModeSelect/1 -> Unit Delay/1
  Unit Delay/1 -> McModeManage/14(WorkStateModeSelectBefore)  "M_State_WorkStateModeSelectBefore_u16"
  WorkCmdAnalog_RunCmd/1 -> WorkCmdJudge/17(WorkCmdAnalog_RunCmd)
  WorkCmdAnalog_ModeCmd/1 -> WorkCmdJudge/1(WorkCmdAnalog_ModeCmd)
  WorkCmdAnalog_TorqueCmd/1 -> WorkCmdJudge/19(WorkCmdAnalog_TorqueCmd)
  WorkCmdAnalog_SpeedCmd/1 -> WorkCmdJudge/18(WorkCmdAnalog_SpeedCmd)
  CurrentPolarCoordinatesFlg/1 -> McModeManage/11(CurrentPolarCoordinatesFlg)
  ZeroTorqueFlag/1 -> McModeManage/12(ZeroTorqueFlag)
  SpeedCal_speed2ms/1 -> McModeManage/13(SpeedCal_speed2ms)
  McModeManage/10(SpeedCtrl_SpeedCmdFilter) -> SpeedCtrl_SpeedCmdFilter/1  "M_State_SpeedCtrlCmdFilter_s32"

== system MCU_Stateflow_Analog/Task_2ms/草稿 ==
  Chart : Stateflow chart  Commented=on  TreatAsAtomicUnit=on
      settings: PortSchema="{\"entries\":[{\"content\":{\"sides\":[{\"content\":{\"connectorIds\":[\"In2\",\"In4\",\"In3\",\"In5\",\"In6\",\"In7\",\"In8\",\"In9\",\"In10\",\"In11\",\"In1\"]},\"type\":\"ConnectorPlacement.EquallySpacedRectSide\",\"uuid\":\"2e7d3842-0a61-4590-9292-7a5bc1b6d63e\"},{\"content\":{\"connectorIds\":[\"Out1\",\"Out2\",\"Out3\",\"Out4\",\"Out5\",\"Out6\",\"Out7\",\"Out8\",\"Out9\"],\"side\":\"RIGHT\"},\"type\":\"ConnectorPlacement.EquallySpacedRectSide\",\"uuid\":\"fb66f02a-321f-47a6-a489-4b94442e22c8\"},{\"content\":{\"connectorIds\":[],\"side\":\"TOP\"},\"type\":\"ConnectorPlacement.EquallySpacedRectSide\",\"uuid\":\"26cfdcf8-827e-48d9-aa42-40739db869be\"},{\"content\":{\"connectorIds\":[],\"side\":\"BOTTOM\"},\"type\":\"ConnectorPlacement.EquallySpacedRectSide\",\"uuid\":\"3bc2be8d-756f-48d1-976e-919451ea6fa2\"}]},\"type\":\"ConnectorPlacement.EquallySpacedConnector\",\"uuid\":\"eb156a25-beb1-4594-a414-e9203ec852c3\"}],\"packageUris\":[\"http://schema.mathworks.com/mf0/Connector/R2020b\"],\"version\":\"1.0\"}"
  Chart2 : Stateflow chart  Commented=on  TreatAsAtomicUnit=on
      settings: PortSchema="{\"entries\":[{\"content\":{\"sides\":[{\"content\":{\"connectorIds\":[\"In2\",\"In4\",\"In3\",\"In5\",\"In6\",\"In7\",\"In8\",\"In9\",\"In10\",\"In1\",\"In11\"]},\"type\":\"ConnectorPlacement.EquallySpacedRectSide\",\"uuid\":\"2e7d3842-0a61-4590-9292-7a5bc1b6d63e\"},{\"content\":{\"connectorIds\":[\"Out1\",\"Out2\",\"Out3\",\"Out4\",\"Out5\",\"Out6\",\"Out7\",\"Out8\",\"Out9\"],\"side\":\"RIGHT\"},\"type\":\"ConnectorPlacement.EquallySpacedRectSide\",\"uuid\":\"fb66f02a-321f-47a6-a489-4b94442e22c8\"},{\"content\":{\"connectorIds\":[],\"side\":\"TOP\"},\"type\":\"ConnectorPlacement.EquallySpacedRectSide\",\"uuid\":\"26cfdcf8-827e-48d9-aa42-40739db869be\"},{\"content\":{\"connectorIds\":[],\"side\":\"BOTTOM\"},\"type\":\"ConnectorPlacement.EquallySpacedRectSide\",\"uuid\":\"3bc2be8d-756f-48d1-976e-919451ea6fa2\"}]},\"type\":\"ConnectorPlacement.EquallySpacedConnector\",\"uuid\":\"eb156a25-beb1-4594-a414-e9203ec852c3\"}],\"packageUris\":[\"http://schema.mathworks.com/mf0/Connector/R2020b\"],\"version\":\"1.0\"}"
  MotorState1 : Stateflow chart  Commented=on  TreatAsAtomicUnit=on
  MotorState2 : Stateflow chart  Commented=on  TreatAsAtomicUnit=on
      settings: PortSchema="{\"entries\":[{\"content\":{\"sides\":[{\"content\":{\"connectorIds\":[\"In12\",\"In7\",\"In8\",\"In9\",\"In10\",\"In11\",\"In13\",\"In14\",\"In6\",\"In15\",\"In5\",\"In4\",\"In3\",\"In2\",\"In1\"]},\"type\":\"ConnectorPlacement.EquallySpacedRectSide\",\"uuid\":\"e0adab7d-9c82-44fd-b38c-331bb9d71454\"},{\"content\":{\"connectorIds\":[\"Out1\",\"Out2\",\"Out3\"],\"side\":\"RIGHT\"},\"type\":\"ConnectorPlacement.EquallySpacedRectSide\",\"uuid\":\"98ad1acc-debf-46f0-91aa-4bd2062f60b6\"},{\"content\":{\"connectorIds\":[],\"side\":\"TOP\"},\"type\":\"ConnectorPlacement.EquallySpacedRectSide\",\"uuid\":\"a7c2d312-245c-4ce1-bea5-1bac95c515f1\"},{\"content\":{\"connectorIds\":[],\"side\":\"BOTTOM\"},\"type\":\"ConnectorPlacement.EquallySpacedRectSide\",\"uuid\":\"175f3b6b-1019-4e6e-83d9-bf4c82f74bc8\"}]},\"type\":\"ConnectorPlacement.EquallySpacedConnector\",\"uuid\":\"df312d8c-c57e-4b1a-958b-330641c1b4d1\"}],\"packageUris\":[\"http://schema.mathworks.com/mf0/Connector/R2020b\"],\"version\":\"1.0\"}"
  MotorState3 : Stateflow chart  TreatAsAtomicUnit=on
      settings: PortSchema="{\"entries\":[{\"content\":{\"sides\":[{\"content\":{\"connectorIds\":[\"In5\",\"In1\",\"In2\",\"In3\",\"In4\"]},\"type\":\"ConnectorPlacement.EquallySpacedRectSide\",\"uuid\":\"e0adab7d-9c82-44fd-b38c-331bb9d71454\"},{\"content\":{\"connectorIds\":[\"Out1\",\"Out2\",\"Out3\"],\"side\":\"RIGHT\"},\"type\":\"ConnectorPlacement.EquallySpacedRectSide\",\"uuid\":\"98ad1acc-debf-46f0-91aa-4bd2062f60b6\"},{\"content\":{\"connectorIds\":[],\"side\":\"TOP\"},\"type\":\"ConnectorPlacement.EquallySpacedRectSide\",\"uuid\":\"a7c2d312-245c-4ce1-bea5-1bac95c515f1\"},{\"content\":{\"connectorIds\":[],\"side\":\"BOTTOM\"},\"type\":\"ConnectorPlacement.EquallySpacedRectSide\",\"uuid\":\"175f3b6b-1019-4e6e-83d9-bf4c82f74bc8\"}]},\"type\":\"ConnectorPlacement.EquallySpacedConnector\",\"uuid\":\"df312d8c-c57e-4b1a-958b-330641c1b4d1\"}],\"packageUris\":[\"http://schema.mathworks.com/mf0/Connector/R2020b\"],\"version\":\"1.0\"}"
  MotorState4 : Stateflow chart  Commented=on  TreatAsAtomicUnit=on
      settings: PortSchema="{\"entries\":[{\"content\":{\"sides\":[{\"content\":{\"connectorIds\":[\"In4\",\"In3\",\"In1\",\"In2\",\"In5\"]},\"type\":\"ConnectorPlacement.EquallySpacedRectSide\",\"uuid\":\"e0adab7d-9c82-44fd-b38c-331bb9d71454\"},{\"content\":{\"connectorIds\":[\"Out1\",\"Out2\",\"Out3\"],\"side\":\"RIGHT\"},\"type\":\"ConnectorPlacement.EquallySpacedRectSide\",\"uuid\":\"98ad1acc-debf-46f0-91aa-4bd2062f60b6\"},{\"content\":{\"connectorIds\":[],\"side\":\"TOP\"},\"type\":\"ConnectorPlacement.EquallySpacedRectSide\",\"uuid\":\"a7c2d312-245c-4ce1-bea5-1bac95c515f1\"},{\"content\":{\"connectorIds\":[],\"side\":\"BOTTOM\"},\"type\":\"ConnectorPlacement.EquallySpacedRectSide\",\"uuid\":\"175f3b6b-1019-4e6e-83d9-bf4c82f74bc8\"}]},\"type\":\"ConnectorPlacement.EquallySpacedConnector\",\"uuid\":\"df312d8c-c57e-4b1a-958b-330641c1b4d1\"}],\"packageUris\":[\"http://schema.mathworks.com/mf0/Connector/R2020b\"],\"version\":\"1.0\"}"

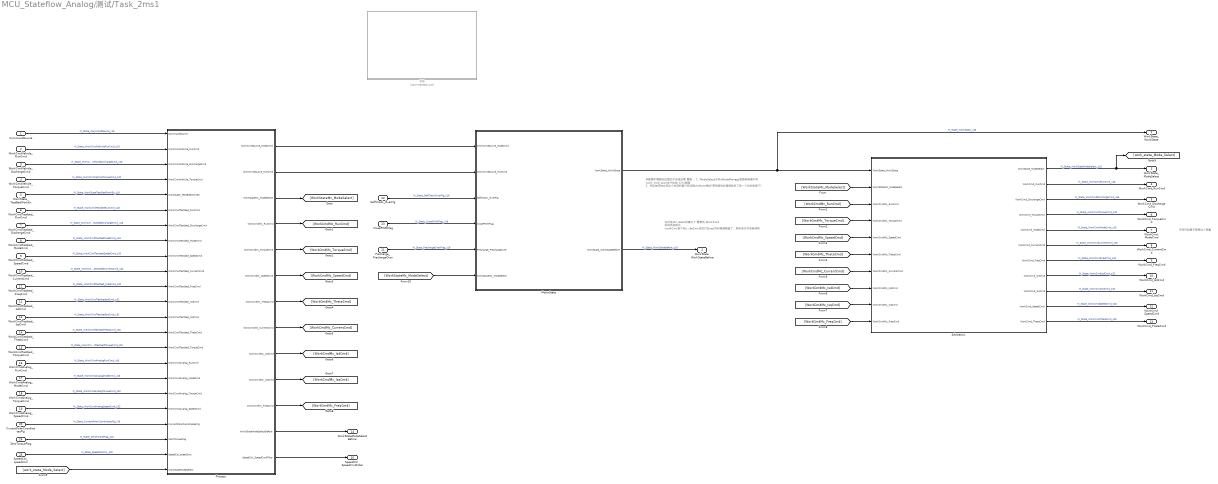
== system MCU_Stateflow_Analog/测试/Task_2ms1 ==
  note: 手写代码里不使用这个变量
  note: 在出现ctrl_reset的情况下
      | 需要将 WorkCmd 的成员初始化
      | workCmd有个ModeCmd成员只在rest的时候被赋值了，其他地方并没有调用
  note: 判断需不需要在后面的子系统处理
      |
      | 需要：
      | 1、ModeSelect在McModeManage里面有根据不同 work_cmd_source.Mode_Cmd赋值
      | 2、ModeSelect在这个状态机里只有切换为cNone模式(零扭矩的处理被放在了前一个状态机里了)
  CommandSource : Inport
  WorkCmdVehicle_RunCmd : Inport  Port=2
  WorkCmdVehicle_DischargeCmd : Inport  Port=3
  WorkCmdVehicle_TorqueCmd : Inport  Port=4
  WorkState_TestBedWorkEn : Inport  Port=5
  WorkCmdTestbed_RunCmd : Inport  Port=6
  WorkCmdTestbed_DischargeCmd : Inport  Port=7
  WorkCmdTestbed_ModeCmd : Inport  Port=8
  WorkCmdTestbed_SpeedCmd : Inport  Port=9
  WorkCmdTestbed_CurrentCmd : Inport  Port=10
  WorkCmdTestbed_FreqCmd : Inport  Port=11
  WorkCmdTestbed_IsdCmd : Inport  Port=12
  WorkCmdTestbed_IsqCmd : Inport  Port=13
  WorkCmdTestbed_ThetaCmd : Inport  Port=14
  WorkCmdTestbed_TorqueCmd : Inport  Port=15
  WorkCmdAnalog_RunCmd : Inport  Port=16
  WorkCmdAnalog_ModeCmd : Inport  Port=17
  WorkCmdAnalog_TorqueCmd : Inport  Port=18
  WorkCmdAnalog_SpeedCmd : Inport  Port=19
  CurrentPolarCoordinatesFlg : Inport  Port=20
  Precharge_PrechargeOver : Inport  Port=21
  SelfCheck_OverFlg : Inport  Port=22
  ClosePWMFlag : Inport  Port=23
  ZeroTorqueFlag : Inport  Port=24
  SpeedCal_speed2ms : Inport  Port=25
  Arbitration : Subsystem  TreatAsAtomicUnit=on
      settings: RTWSystemCode=Nonreusable function
  MotorState : Stateflow chart  TreatAsAtomicUnit=on
      settings: RTWSystemCode=Nonreusable function  PortSchema="{\"entries\":[{\"content\":{\"sides\":[{\"content\":{\"connectorIds\":[\"In4\",\"In3\",\"In1\",\"In2\",\"In5\",\"In6\"]},\"type\":\"ConnectorPlacement.EquallySpacedRectSide\",\"uuid\":\"e0adab7d-9c82-44fd-b38c-331bb9d71454\"},{\"content\":{\"connectorIds\":[\"Out1\",\"Out2\"],\"side\":\"RIGHT\"},\"type\":\"ConnectorPlacement.EquallySpacedRectSide\",\"uuid\":\"98ad1acc-debf-46f0-91aa-4bd2062f60b6\"},{\"content\":{\"connectorIds\":[],\"side\":\"TOP\"},\"type\":\"ConnectorPlacement.EquallySpacedRectSide\",\"uuid\":\"a7c2d312-245c-4ce1-bea5-1bac95c515f1\"},{\"content\":{\"connectorIds\":[],\"side\":\"BOTTOM\"},\"type\":\"ConnectorPlacement.EquallySpacedRectSide\",\"uuid\":\"175f3b6b-1019-4e6e-83d9-bf4c82f74bc8\"}]},\"type\":\"ConnectorPlacement.EquallySpacedConnector\",\"uuid\":\"df312d8c-c57e-4b1a-958b-330641c1b4d1\"}],\"packageUris\":[\"http://schema.mathworks.com/mf0/Connector/R2020b\"],\"version\":\"1.0\"}"
  Process : Subsystem  TreatAsAtomicUnit=on
  草稿 : Subsystem  Commented=on
  WorkState_WorkState : Outport
  WorkState_WorkStateBefore : Outport  Port=2
  WorkState_ModeSelect : Outport  Port=3
  WorkCmd_RunCmd : Outport  Port=4
  WorkCmd_DischargeCmd : Outport  Port=5
  WorkCmd_TorqueCmd : Outport  Port=6
  WorkCmd_ModeCmd : Outport  Port=7
  WorkCmd_CurrentCmd : Outport  Port=8
  WorkCmd_FreqCmd : Outport  Port=9
  WorkCmd_IsdCmd : Outport  Port=10
  WorkCmd_IsqCmd : Outport  Port=11
  WorkCmd_SpeedCmd : Outport  Port=12
  WorkCmd_ThetaCmd : Outport  Port=13
  WorkStateModeSelectBefore : Outport  Port=14
  SpeedCtrl_SpeedCmdFilter : Outport  Port=15
  wires:
  MotorState/1(WorkState_WorkState) -> Arbitration/1(WorkState_WorkState), WorkState_WorkState/1  "M_State_WorkState_u16"
  [WorkStateMc_ModeSelect] -> Arbitration/2(WorkStateMc_ModeSelect)
  [WorkCmdMc_RunCmd] -> Arbitration/3(WorkCmdMc_RunCmd)
  [WorkCmdMc_TorqueCmd] -> Arbitration/4(WorkCmdMc_TorqueCmd)
  [WorkCmdMc_SpeedCmd] -> Arbitration/5(WorkCmdMc_SpeedCmd)
  [WorkCmdMc_ThetaCmd] -> Arbitration/6(WorkCmdMc_ThetaCmd)
  [WorkCmdMc_CurrentCmd] -> Arbitration/7(WorkCmdMc_CurrentCmd)
  [WorkCmdMc_IsdCmd] -> Arbitration/8(WorkCmdMc_IsdCmd)
  [WorkCmdMc_IsqCmd] -> Arbitration/9(WorkCmdMc_IsqCmd)
  [WorkCmdMc_FreqCmd] -> Arbitration/10(WorkCmdMc_FreqCmd)
  Precharge_PrechargeOver/1 -> MotorState/5(Precharge_PrechargeOver)  "M_State_PrechargeOverFlag_u16"
  MotorState/2(WorkState_WorkStateBefore) -> WorkState_WorkStateBefore/1  "M_State_WorkStateBefore_u16"
  Process/7(WorkCmdMc_ThetaCmd) -> [WorkCmdMc_ThetaCmd]
  Process/8(WorkCmdMc_CurrentCmd) -> [WorkCmdMc_CurrentCmd]
  Process/6(WorkCmdMc_SpeedCmd) -> [WorkCmdMc_SpeedCmd]
  Process/11(WorkCmdMc_FreqCmd) -> [WorkCmdMc_FreqCmd]
  Process/4(WorkCmdMc_RunCmd) -> [WorkCmdMc_RunCmd]
  Process/9(WorkCmdMc_IsdCmd) -> [WorkCmdMc_IsdCmd]
  Process/10(WorkCmdMc_IsqCmd) -> [WorkCmdMc_IsqCmd]
  Process/5(WorkCmdMc_TorqueCmd) -> [WorkCmdMc_TorqueCmd]
  Process/3(WorkStateMc_ModeSelect) -> [WorkStateMc_ModeSelect]
  CommandSource/1 -> Process/1(CommandSource)  "M_State_CommandSource_i16"
  WorkCmdVehicle_RunCmd/1 -> Process/2(WorkCmdVehicle_RunCmd)  "M_State_WorkCmdVehicleRunCmd_u16"
  WorkCmdVehicle_DischargeCmd/1 -> Process/3(WorkCmdVehicle_DischargeCmd)  "M_State_WorkCmdVehicleDischargeCmd_u16"
  WorkState_TestBedWorkEn/1 -> Process/5(WorkState_TestBedWorkEn)  "M_State_WorkStateTestBedWorkEn_u16"
  WorkCmdTestbed_RunCmd/1 -> Process/6(WorkCmdTestbed_RunCmd)  "M_State_WorkCmdTestbedRunCmd_u16"
  WorkCmdTestbed_DischargeCmd/1 -> Process/7(WorkCmdTestbed_DischargeCmd)  "M_State_WorkCmdTestbedDischargeCmd_u16"
  WorkCmdTestbed_ModeCmd/1 -> Process/8(WorkCmdTestbed_ModeCmd)  "M_State_WorkCmdTestbedModeCmd_u16"
  WorkCmdTestbed_SpeedCmd/1 -> Process/9(WorkCmdTestbed_SpeedCmd)  "M_State_WorkCmdTestbedSpeedCmd_s32"
  WorkCmdTestbed_CurrentCmd/1 -> Process/10(WorkCmdTestbed_CurrentCmd)  "M_State_WorkCmdTestbedCurrentCmd_s32"
  WorkCmdTestbed_FreqCmd/1 -> Process/11(WorkCmdTestbed_FreqCmd)  "M_State_WorkCmdTestbed_FreqCmd_s32"
  WorkCmdTestbed_IsdCmd/1 -> Process/12(WorkCmdTestbed_IsdCmd)  "M_State_WorkCmdTestbedIsdCmd_s32"
  WorkCmdTestbed_IsqCmd/1 -> Process/13(WorkCmdTestbed_IsqCmd)  "M_State_WorkCmdTestbedIsqCmd_s32"
  WorkCmdTestbed_ThetaCmd/1 -> Process/14(WorkCmdTestbed_ThetaCmd)  "M_State_WorkCmdTestbedThetaCmd_s32"
  WorkCmdVehicle_TorqueCmd/1 -> Process/4(WorkCmdVehicle_TorqueCmd)  "M_State_WorkCmdVehicleTorqueCmd_s32"
  WorkCmdTestbed_TorqueCmd/1 -> Process/15(WorkCmdTestbed_TorqueCmd)  "M_State_WorkCmdTestbedTorqueCmd_s32"
  CurrentPolarCoordinatesFlg/1 -> Process/20(CurrentPolarCoordinatesFlg)  "M_State_CurrentPolarCoordinatesFlg_i16"
  ZeroTorqueFlag/1 -> Process/21(ZeroTorqueFlag)  "M_State_ZeroTorqueFlag_u16"
  Process/1(WorkCmdSource_ModeCmd) -> MotorState/4(WorkCmdSource_ModeCmd)
  Process/2(WorkCmdSource_RunCmd) -> MotorState/3(WorkCmdSource_RunCmd)
  Arbitration/1(WorkState_ModeSelect) -> WorkState_ModeSelect/1, [work_state_Mode_Select]  "M_State_WorkStateModeSelect_u16"
  Arbitration/2(WorkCmd_RunCmd) -> WorkCmd_RunCmd/1  "M_State_WorkCmdRunCmd_u16"
  Arbitration/3(WorkCmd_DischargeCmd) -> WorkCmd_DischargeCmd/1  "M_State_WorkCmdDischargeCmd_u16"
  Arbitration/4(WorkCmd_TorqueCmd) -> WorkCmd_TorqueCmd/1  "M_State_WorkCmdTorqueCmd_s32"
  Arbitration/5(WorkCmd_ModeCmd) -> WorkCmd_ModeCmd/1  "M_State_WorkCmdModeCmd_u16"
  Arbitration/6(WorkCmd_CurrentCmd) -> WorkCmd_CurrentCmd/1  "M_State_WorkCmdCurrentCmd_s32"
  Arbitration/7(WorkCmd_FreqCmd) -> WorkCmd_FreqCmd/1  "M_State_WorkCmdFreqCmd_s32"
  Arbitration/8(WorkCmd_IsdCmd) -> WorkCmd_IsdCmd/1  "M_State_WorkCmdIsdCmd_s32"
  Arbitration/9(WorkCmd_IsqCmd) -> WorkCmd_IsqCmd/1  "M_State_WorkCmdIsqCmd_s32"
  Arbitration/10(WorkCmd_SpeedCmd) -> WorkCmd_SpeedCmd/1  "M_State_WorkCmdSpeedCmd_s32"
  Arbitration/11(WorkCmd_ThetaCmd) -> WorkCmd_ThetaCmd/1  "M_State_WorkCmdThetaCmd_s32"
  SelfCheck_OverFlg/1 -> MotorState/1(SelfCheck_OverFlg)  "M_State_SelfCheckOverFlg_u16"
  ClosePWMFlag/1 -> MotorState/2(ClosePWMFlag)  "M_State_ClosePWMFlag_u16"
  [work_state_Mode_Select] -> Process/23(WorkStateModeSelect)
  [WorkStateMc_ModeSelect] -> MotorState/6(WorkStateMc_ModeSelect)
  Process/12(WorkStateModeSelectBefore) -> WorkStateModeSelectBefore/1
  WorkCmdAnalog_RunCmd/1 -> Process/16(WorkCmdAnalog_RunCmd)  "M_State_WorkCmdAnalogRunCmd_u16"
  WorkCmdAnalog_ModeCmd/1 -> Process/17(WorkCmdAnalog_ModeCmd)  "M_State_WorkCmdAnalogModeCmd_u16"
  WorkCmdAnalog_TorqueCmd/1 -> Process/18(WorkCmdAnalog_TorqueCmd)  "M_State_WorkCmdAnalogTorqueCmd_s32"
  WorkCmdAnalog_SpeedCmd/1 -> Process/19(WorkCmdAnalog_SpeedCmd)  "M_State_WorkCmdAnalogSpeedCmd_s32"
  SpeedCal_speed2ms/1 -> Process/22(SpeedCal_speed2ms)  "M_State_SpeedCal2ms_s32"
  Process/13(SpeedCtrl_SpeedCmdFilter) -> SpeedCtrl_SpeedCmdFilter/1

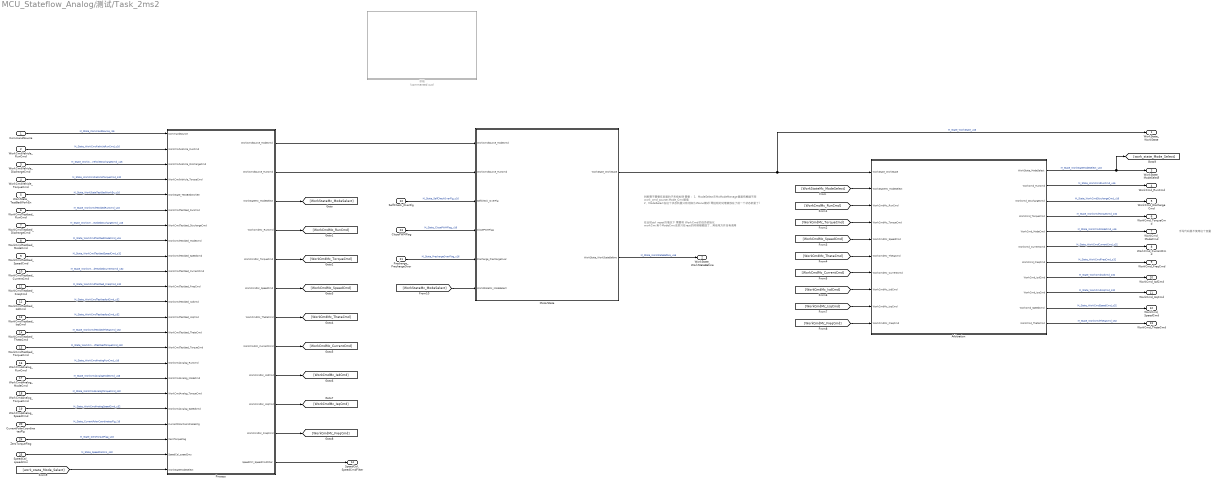
== system MCU_Stateflow_Analog/测试/Task_2ms2 ==
  note: 手写代码里不使用这个变量
  note: 在出现ctrl_reset的情况下
      | 需要将 WorkCmd 的成员初始化
      | workCmd有个ModeCmd成员只在rest的时候被赋值了，其他地方并没有调用
  note: 判断需不需要在后面的子系统处理
      |
      | 需要：
      | 1、ModeSelect在McModeManage里面有根据不同 work_cmd_source.Mode_Cmd赋值
      | 2、ModeSelect在这个状态机里只有切换为cNone模式(零扭矩的处理被放在了前一个状态机里了)
  CommandSource : Inport
  WorkCmdVehicle_RunCmd : Inport  Port=2
  WorkCmdVehicle_DischargeCmd : Inport  Port=3
  WorkCmdVehicle_TorqueCmd : Inport  Port=4
  WorkState_TestBedWorkEn : Inport  Port=5
  WorkCmdTestbed_RunCmd : Inport  Port=6
  WorkCmdTestbed_DischargeCmd : Inport  Port=7
  WorkCmdTestbed_ModeCmd : Inport  Port=8
  WorkCmdTestbed_SpeedCmd : Inport  Port=9
  WorkCmdTestbed_CurrentCmd : Inport  Port=10
  WorkCmdTestbed_FreqCmd : Inport  Port=11
  WorkCmdTestbed_IsdCmd : Inport  Port=12
  WorkCmdTestbed_IsqCmd : Inport  Port=13
  WorkCmdTestbed_ThetaCmd : Inport  Port=14
  WorkCmdTestbed_TorqueCmd : Inport  Port=15
  WorkCmdAnalog_RunCmd : Inport  Port=16
  WorkCmdAnalog_ModeCmd : Inport  Port=17
  WorkCmdAnalog_TorqueCmd : Inport  Port=18
  WorkCmdAnalog_SpeedCmd : Inport  Port=19
  CurrentPolarCoordinatesFlg : Inport  Port=20
  Precharge_PrechargeOver : Inport  Port=21
  SelfCheck_OverFlg : Inport  Port=22
  ClosePWMFlag : Inport  Port=23
  ZeroTorqueFlag : Inport  Port=24
  SpeedCal_speed2ms : Inport  Port=25
  Arbitration : Subsystem  TreatAsAtomicUnit=on
      settings: RTWSystemCode=Nonreusable function
  MotorState : Stateflow chart
      settings: RTWSystemCode=Reusable function  PortSchema="{\"entries\":[{\"content\":{\"sides\":[{\"content\":{\"connectorIds\":[\"In4\",\"In3\",\"In1\",\"In2\",\"In5\",\"In6\"]},\"type\":\"ConnectorPlacement.EquallySpacedRectSide\",\"uuid\":\"e0adab7d-9c82-44fd-b38c-331bb9d71454\"},{\"content\":{\"connectorIds\":[\"Out1\",\"Out2\"],\"side\":\"RIGHT\"},\"type\":\"ConnectorPlacement.EquallySpacedRectSide\",\"uuid\":\"98ad1acc-debf-46f0-91aa-4bd2062f60b6\"},{\"content\":{\"connectorIds\":[],\"side\":\"TOP\"},\"type\":\"ConnectorPlacement.EquallySpacedRectSide\",\"uuid\":\"a7c2d312-245c-4ce1-bea5-1bac95c515f1\"},{\"content\":{\"connectorIds\":[],\"side\":\"BOTTOM\"},\"type\":\"ConnectorPlacement.EquallySpacedRectSide\",\"uuid\":\"175f3b6b-1019-4e6e-83d9-bf4c82f74bc8\"}]},\"type\":\"ConnectorPlacement.EquallySpacedConnector\",\"uuid\":\"df312d8c-c57e-4b1a-958b-330641c1b4d1\"}],\"packageUris\":[\"http://schema.mathworks.com/mf0/Connector/R2020b\"],\"version\":\"1.0\"}"
  Process : Subsystem  TreatAsAtomicUnit=on
  草稿 : Subsystem  Commented=on
  WorkState_WorkState : Outport
  WorkState_WorkStateBefore : Outport  Port=2
  WorkState_ModeSelect : Outport  Port=3
  WorkCmd_RunCmd : Outport  Port=4
  WorkCmd_DischargeCmd : Outport  Port=5
  WorkCmd_TorqueCmd : Outport  Port=6
  WorkCmd_ModeCmd : Outport  Port=7
  WorkCmd_CurrentCmd : Outport  Port=8
  WorkCmd_FreqCmd : Outport  Port=9
  WorkCmd_IsdCmd : Outport  Port=10
  WorkCmd_IsqCmd : Outport  Port=11
  WorkCmd_SpeedCmd : Outport  Port=12
  WorkCmd_ThetaCmd : Outport  Port=13
  SpeedCtrl_SpeedCmdFilter : Outport  Port=14
  wires:
  MotorState/1(WorkState_WorkState) -> WorkState_WorkState/1, Arbitration/1(WorkState_WorkState)  "M_State_WorkState_u16"
  [WorkStateMc_ModeSelect] -> Arbitration/2(WorkStateMc_ModeSelect)
  [WorkCmdMc_RunCmd] -> Arbitration/3(WorkCmdMc_RunCmd)
  [WorkCmdMc_TorqueCmd] -> Arbitration/4(WorkCmdMc_TorqueCmd)
  [WorkCmdMc_SpeedCmd] -> Arbitration/5(WorkCmdMc_SpeedCmd)
  [WorkCmdMc_ThetaCmd] -> Arbitration/6(WorkCmdMc_ThetaCmd)
  [WorkCmdMc_CurrentCmd] -> Arbitration/7(WorkCmdMc_CurrentCmd)
  [WorkCmdMc_IsdCmd] -> Arbitration/8(WorkCmdMc_IsdCmd)
  [WorkCmdMc_IsqCmd] -> Arbitration/9(WorkCmdMc_IsqCmd)
  [WorkCmdMc_FreqCmd] -> Arbitration/10(WorkCmdMc_FreqCmd)
  Precharge_PrechargeOver/1 -> MotorState/5(Precharge_PrechargeOver)  "M_State_PrechargeOverFlag_u16"
  MotorState/2(WorkState_WorkStateBefore) -> WorkState_WorkStateBefore/1  "M_State_WorkStateBefore_u16"
  Process/7(WorkCmdMc_ThetaCmd) -> [WorkCmdMc_ThetaCmd]
  Process/8(WorkCmdMc_CurrentCmd) -> [WorkCmdMc_CurrentCmd]
  Process/6(WorkCmdMc_SpeedCmd) -> [WorkCmdMc_SpeedCmd]
  Process/11(WorkCmdMc_FreqCmd) -> [WorkCmdMc_FreqCmd]
  Process/4(WorkCmdMc_RunCmd) -> [WorkCmdMc_RunCmd]
  Process/9(WorkCmdMc_IsdCmd) -> [WorkCmdMc_IsdCmd]
  Process/10(WorkCmdMc_IsqCmd) -> [WorkCmdMc_IsqCmd]
  Process/5(WorkCmdMc_TorqueCmd) -> [WorkCmdMc_TorqueCmd]
  Process/3(WorkStateMc_ModeSelect) -> [WorkStateMc_ModeSelect]
  CommandSource/1 -> Process/1(CommandSource)  "M_State_CommandSource_i16"
  WorkCmdVehicle_RunCmd/1 -> Process/2(WorkCmdVehicle_RunCmd)  "M_State_WorkCmdVehicleRunCmd_u16"
  WorkCmdVehicle_DischargeCmd/1 -> Process/3(WorkCmdVehicle_DischargeCmd)  "M_State_WorkCmdVehicleDischargeCmd_u16"
  WorkState_TestBedWorkEn/1 -> Process/5(WorkState_TestBedWorkEn)  "M_State_WorkStateTestBedWorkEn_u16"
  WorkCmdTestbed_RunCmd/1 -> Process/6(WorkCmdTestbed_RunCmd)  "M_State_WorkCmdTestbedRunCmd_u16"
  WorkCmdTestbed_DischargeCmd/1 -> Process/7(WorkCmdTestbed_DischargeCmd)  "M_State_WorkCmdTestbedDischargeCmd_u16"
  WorkCmdTestbed_ModeCmd/1 -> Process/8(WorkCmdTestbed_ModeCmd)  "M_State_WorkCmdTestbedModeCmd_u16"
  WorkCmdTestbed_SpeedCmd/1 -> Process/9(WorkCmdTestbed_SpeedCmd)  "M_State_WorkCmdTestbedSpeedCmd_s32"
  WorkCmdTestbed_CurrentCmd/1 -> Process/10(WorkCmdTestbed_CurrentCmd)  "M_State_WorkCmdTestbedCurrentCmd_s32"
  WorkCmdTestbed_FreqCmd/1 -> Process/11(WorkCmdTestbed_FreqCmd)  "M_State_WorkCmdTestbed_FreqCmd_s32"
  WorkCmdTestbed_IsdCmd/1 -> Process/12(WorkCmdTestbed_IsdCmd)  "M_State_WorkCmdTestbedIsdCmd_s32"
  WorkCmdTestbed_IsqCmd/1 -> Process/13(WorkCmdTestbed_IsqCmd)  "M_State_WorkCmdTestbedIsqCmd_s32"
  WorkCmdTestbed_ThetaCmd/1 -> Process/14(WorkCmdTestbed_ThetaCmd)  "M_State_WorkCmdTestbedThetaCmd_s32"
  WorkCmdVehicle_TorqueCmd/1 -> Process/4(WorkCmdVehicle_TorqueCmd)  "M_State_WorkCmdVehicleTorqueCmd_s32"
  WorkCmdTestbed_TorqueCmd/1 -> Process/15(WorkCmdTestbed_TorqueCmd)  "M_State_WorkCmdTestbedTorqueCmd_s32"
  CurrentPolarCoordinatesFlg/1 -> Process/20(CurrentPolarCoordinatesFlg)  "M_State_CurrentPolarCoordinatesFlg_i16"
  ZeroTorqueFlag/1 -> Process/21(ZeroTorqueFlag)  "M_State_ZeroTorqueFlag_u16"
  Process/1(WorkCmdSource_ModeCmd) -> MotorState/4(WorkCmdSource_ModeCmd)
  Process/2(WorkCmdSource_RunCmd) -> MotorState/3(WorkCmdSource_RunCmd)
  Arbitration/1(WorkState_ModeSelect) -> WorkState_ModeSelect/1, [work_state_Mode_Select]  "M_State_WorkStateModeSelect_u16"
  Arbitration/2(WorkCmd_RunCmd) -> WorkCmd_RunCmd/1  "M_State_WorkCmdRunCmd_u16"
  Arbitration/3(WorkCmd_DischargeCmd) -> WorkCmd_DischargeCmd/1  "M_State_WorkCmdDischargeCmd_u16"
  Arbitration/4(WorkCmd_TorqueCmd) -> WorkCmd_TorqueCmd/1  "M_State_WorkCmdTorqueCmd_s32"
  Arbitration/5(WorkCmd_ModeCmd) -> WorkCmd_ModeCmd/1  "M_State_WorkCmdModeCmd_u16"
  Arbitration/6(WorkCmd_CurrentCmd) -> WorkCmd_CurrentCmd/1  "M_State_WorkCmdCurrentCmd_s32"
  Arbitration/7(WorkCmd_FreqCmd) -> WorkCmd_FreqCmd/1  "M_State_WorkCmdFreqCmd_s32"
  Arbitration/8(WorkCmd_IsdCmd) -> WorkCmd_IsdCmd/1  "M_State_WorkCmdIsdCmd_s32"
  Arbitration/9(WorkCmd_IsqCmd) -> WorkCmd_IsqCmd/1  "M_State_WorkCmdIsqCmd_s32"
  Arbitration/10(WorkCmd_SpeedCmd) -> WorkCmd_SpeedCmd/1  "M_State_WorkCmdSpeedCmd_s32"
  Arbitration/11(WorkCmd_ThetaCmd) -> WorkCmd_ThetaCmd/1  "M_State_WorkCmdThetaCmd_s32"
  SelfCheck_OverFlg/1 -> MotorState/1(SelfCheck_OverFlg)  "M_State_SelfCheckOverFlg_u16"
  ClosePWMFlag/1 -> MotorState/2(ClosePWMFlag)  "M_State_ClosePWMFlag_u16"
  [work_state_Mode_Select] -> Process/23(WorkStateModeSelect)
  [WorkStateMc_ModeSelect] -> MotorState/6(WorkStateMc_ModeSelect)
  WorkCmdAnalog_RunCmd/1 -> Process/16(WorkCmdAnalog_RunCmd)  "M_State_WorkCmdAnalogRunCmd_u16"
  WorkCmdAnalog_ModeCmd/1 -> Process/17(WorkCmdAnalog_ModeCmd)  "M_State_WorkCmdAnalogModeCmd_u16"
  WorkCmdAnalog_TorqueCmd/1 -> Process/18(WorkCmdAnalog_TorqueCmd)  "M_State_WorkCmdAnalogTorqueCmd_s32"
  WorkCmdAnalog_SpeedCmd/1 -> Process/19(WorkCmdAnalog_SpeedCmd)  "M_State_WorkCmdAnalogSpeedCmd_s32"
  SpeedCal_speed2ms/1 -> Process/22(SpeedCal_speed2ms)  "M_State_SpeedCal2ms_s32"
  Process/12(SpeedCtrl_SpeedCmdFilter) -> SpeedCtrl_SpeedCmdFilter/1
